simulink model "power_grid"  (R2025a)
settings: Solver=VariableStepAuto  StartTime=0.0  StopTime=10.0  RelTol=1e-3
model workspace (MAT data in the model file):
  HPD_1min = 0
values from neighbouring files (symbols this model uses):
  bus_voltage = 230e3    (= 230000)    [initialise.m]
  wind_farm_power = 150e6    (= 150000000)    [initialise.m]
libraries: spsThreePhasePISectionLineLib x7, spsThreePhaseBreakerLib x7, simulink x6, spsThreePhaseVIMeasurementLib x5, spsLoadFlowBusLib x5, spsThreePhaseSeriesRLCLoadLib x4, spsThreePhaseSourceLib x2, spsWindTurbineInductionGeneratorPhasorTypeLib x1, sps_lib x1
settings Model: Creator=pavan  LastModifiedBy=jamim

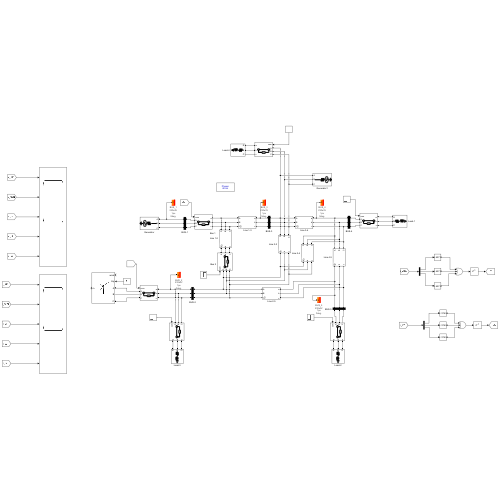
[thumbnail: Simulink's stored preview of the top-level diagram]
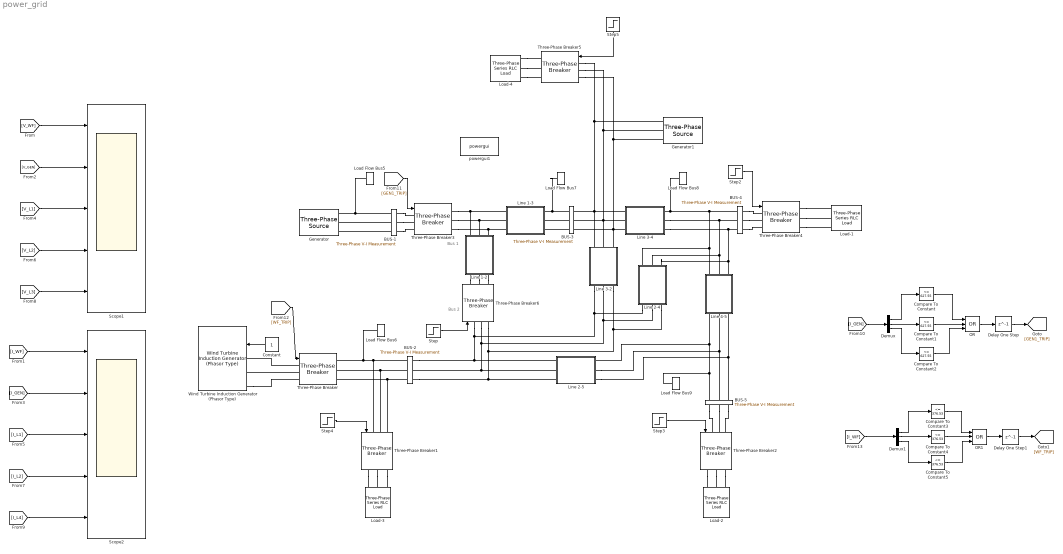
== system power_grid ==
  note: Bus 2
  note: Bus 1
  " Line 1-2" : Subsystem  mask{F=60, SB=100e6, V=230e3, R=0.02, X=0.06, B=0.03}
      mask prompts: F "Frequency"; SB "Base power"; V "Nominal Voltage"; R "Resistance(pu)"; X "Reactance(pu)"; B "Line Charging"
  " Line 1-3" : Subsystem  mask{F=60, SB=100e6, V=230e3, R=0.08, X=0.24, B=0.025}
      mask prompts: F "Frequency"; SB "Base power"; V "Nominal Voltage"; R "Resistance(pu)"; X "Reactance(pu)"; B "Line Charging"
  " Line 2-4" : Subsystem  mask{F=60, SB=100e6, V=230e3, R=0.06, X=0.18, B=0.02}
      mask prompts: F "Frequency"; SB "Base power"; V "Nominal Voltage"; R "Resistance(pu)"; X "Reactance(pu)"; B "Line Charging"
  " Line 2-5" : Subsystem  mask{F=60, SB=100e6, V=230e3, R=0.04, X=0.12, B=0.015}
      mask prompts: F "Frequency"; SB "Base power"; V "Nominal Voltage"; R "Resistance(pu)"; X "Reactance(pu)"; B "Line Charging"
  " Line 3-2" : Subsystem  mask{F=60, SB=100e6, V=230e3, R=0.06, X=0.25, B=0.20}
      mask prompts: F "Frequency"; SB "Base power"; V "Nominal Voltage"; R "Resistance(pu)"; X "Reactance(pu)"; B "Line Charging"
  " Line 3-4" : Subsystem  mask{F=60, SB=100e6, V=230e3, R=0.01, X=0.03, B=0.01}
      mask prompts: F "Frequency"; SB "Base power"; V "Nominal Voltage"; R "Resistance(pu)"; X "Reactance(pu)"; B "Line Charging"
  " Line 4-5" : Subsystem  mask{F=60, SB=100e6, V=230e3, R=0.08, X=0.24, B=0.025}
      mask prompts: F "Frequency"; SB "Base power"; V "Nominal Voltage"; R "Resistance(pu)"; X "Reactance(pu)"; B "Line Charging"
  BUS-1 : spsThreePhaseVIMeasurementLib/Three-Phase V-I Measurement  VoltageMeasurement=phase-to-ground  SetLabelV=on  LabelV=V_GEN  Vpu=off  VpuLL=off  CurrentMeasurement=yes  SetLabelI=on  LabelI=I_GEN  Ipu=off  Pbase=100e6  Vbase=500e3  OutputType=Magnitude  PhasorSimulation=on  PSBequivalent=0
  BUS-2 : spsThreePhaseVIMeasurementLib/Three-Phase V-I Measurement  VoltageMeasurement=phase-to-ground  SetLabelV=on  LabelV=V_WF  Vpu=off  VpuLL=off  CurrentMeasurement=yes  SetLabelI=on  LabelI=I_WF  Ipu=off  Pbase=100e6  Vbase=500e3  OutputType=Magnitude  PhasorSimulation=on  PSBequivalent=0
  BUS-3 : spsThreePhaseVIMeasurementLib/Three-Phase V-I Measurement  VoltageMeasurement=no  SetLabelV=off  LabelV=Vabc  Vpu=off  VpuLL=off  CurrentMeasurement=no  SetLabelI=off  LabelI=Iabc  Ipu=off  Pbase=100e6  Vbase=500e3  OutputType=Complex  PhasorSimulation=on  PSBequivalent=0
  BUS-4 : spsThreePhaseVIMeasurementLib/Three-Phase V-I Measurement  VoltageMeasurement=phase-to-ground  SetLabelV=on  LabelV=V_L1  Vpu=off  VpuLL=off  CurrentMeasurement=yes  SetLabelI=on  LabelI=I_L1  Ipu=off  Pbase=100e6  Vbase=500e3  OutputType=Magnitude  PhasorSimulation=on  PSBequivalent=0
  BUS-5 : spsThreePhaseVIMeasurementLib/Three-Phase V-I Measurement  VoltageMeasurement=phase-to-ground  SetLabelV=on  LabelV=V_L2  Vpu=off  VpuLL=off  CurrentMeasurement=yes  SetLabelI=on  LabelI=I_L2  Ipu=off  Pbase=100e6  Vbase=500e3  OutputType=Magnitude  PhasorSimulation=on  PSBequivalent=0
  Compare To Constant : simulink/Logic and Bit Operations/Compare To Constant  relop=<=  const=627.55  OutDataTypeStr=boolean
  Compare To Constant1 : simulink/Logic and Bit Operations/Compare To Constant  relop=<=  const=627.55  OutDataTypeStr=boolean
  Compare To Constant2 : simulink/Logic and Bit Operations/Compare To Constant  relop=<=  const=627.55  OutDataTypeStr=boolean
  Compare To Constant3 : simulink/Logic and Bit Operations/Compare To Constant  relop=<=  const=376.53  OutDataTypeStr=boolean
  Compare To Constant4 : simulink/Logic and Bit Operations/Compare To Constant  relop=<=  const=376.53  OutDataTypeStr=boolean
  Compare To Constant5 : simulink/Logic and Bit Operations/Compare To Constant  relop=<=  const=376.53  OutDataTypeStr=boolean
  Constant : Constant
  Delay One Step : Delay  DelayLength=1
  Delay One Step1 : Delay  DelayLength=1
  Demux : Demux  Outputs=3
  Demux1 : Demux  Outputs=3
  Generator : spsThreePhaseSourceLib/Three-Phase Source  InternalConnection=Yg  VoltagePhases=off  Voltage=1.06*bus_voltage  PhaseAngle=0  Voltage_phases=[25e3 25e3 25e3]/sqrt(3)  PhaseAngles_phases=[0 -120 +120]  Frequency=60  NonIdealSource=on  SpecifyImpedance=off  Resistance=1e-6  Inductance=0  ShortCircuitLevel=100e6  BaseVoltage=bus_voltage  XRratio=7  BusType=swing  Pref=generator_power  Qref=0  Prefabc=[10e3, 10e3, 10e3]  Qrefabc=[0, 0, 0]  Qmin=-inf  Qmax=inf
  Generator1 : spsThreePhaseSourceLib/Three-Phase Source  InternalConnection=Yg  VoltagePhases=off  Voltage=1.02*bus_voltage  PhaseAngle=0  Voltage_phases=[25e3 25e3 25e3]/sqrt(3)  PhaseAngles_phases=[0 -120 +120]  Frequency=60  NonIdealSource=on  SpecifyImpedance=off  Resistance=1e-6  Inductance=0  ShortCircuitLevel=100e6  BaseVoltage=bus_voltage  XRratio=7  BusType=PV  Pref=generator_power  Qref=0  Prefabc=[10e3, 10e3, 10e3]  Qrefabc=[0, 0, 0]  Qmin=-inf  Qmax=inf
  Load Flow Bus5 : spsLoadFlowBusLib/Load Flow Bus  LConnTagsString=a  Phases=single  Connectors=on one side  ID=BUS_1  Vbase=230e3  Vref=1.06  Vangle=0  VLF=1  VLFb=1  VLFc=1  angleLF=0  angleLFb=0  angleLFc=0
  Load Flow Bus6 : spsLoadFlowBusLib/Load Flow Bus  LConnTagsString=a  Phases=single  Connectors=on one side  ID=BUS_2  Vbase=230e3  Vref=1  Vangle=0  VLF=1  VLFb=1  VLFc=1  angleLF=0  angleLFb=0  angleLFc=0
  Load Flow Bus7 : spsLoadFlowBusLib/Load Flow Bus  LConnTagsString=a  Phases=single  Connectors=on one side  ID=BUS_3  Vbase=230e3  Vref=1  Vangle=0  VLF=1  VLFb=1  VLFc=1  angleLF=0  angleLFb=0  angleLFc=0
  Load Flow Bus8 : spsLoadFlowBusLib/Load Flow Bus  LConnTagsString=a  Phases=single  Connectors=on one side  ID=BUS_4  Vbase=230e3  Vref=1  Vangle=0  VLF=1  VLFb=1  VLFc=1  angleLF=0  angleLFb=0  angleLFc=0
  Load Flow Bus9 : spsLoadFlowBusLib/Load Flow Bus  LConnTagsString=a  Phases=single  Connectors=on one side  ID=BUS_5  Vbase=230e3  Vref=1  Vangle=0  VLF=1  VLFb=1  VLFc=1  angleLF=0  angleLFb=0  angleLFc=0
  Load-1 : spsThreePhaseSeriesRLCLoadLib/Three-Phase Series RLC Load  LConnTagsString=A|B|C  Configuration=Y (grounded)  NominalVoltage=230e3  Vabc=[1e3 1e3 1e3]  Vabcp=[1e3 1e3 1e3]  NominalFrequency=60  UnbalancedPower=off  ActivePower=40e6  InductivePower=20e6  CapacitivePower=0  Pabc=[10e3 9e3 11e3]  QLabc=[100 90 110]  QCabc=[100 90 110]  Pabcp=[10e3 9e3 11e3]  QLabcp=[100 90 110]  QCabcp=[100 90 110]  Measurements=None  LoadType=constant PQ
  Load-2 : spsThreePhaseSeriesRLCLoadLib/Three-Phase Series RLC Load  LConnTagsString=A|B|C  Configuration=Y (grounded)  NominalVoltage=230e3  Vabc=[1e3 1e3 1e3]  Vabcp=[1e3 1e3 1e3]  NominalFrequency=60  UnbalancedPower=off  ActivePower=30e6  InductivePower=15e6  CapacitivePower=0  Pabc=[10e3 9e3 11e3]  QLabc=[100 90 110]  QCabc=[100 90 110]  Pabcp=[10e3 9e3 11e3]  QLabcp=[100 90 110]  QCabcp=[100 90 110]  Measurements=None  LoadType=constant PQ
  Load-3 : spsThreePhaseSeriesRLCLoadLib/Three-Phase Series RLC Load  LConnTagsString=A|B|C  Configuration=Y (grounded)  NominalVoltage=230e3  Vabc=[1e3 1e3 1e3]  Vabcp=[1e3 1e3 1e3]  NominalFrequency=60  UnbalancedPower=off  ActivePower=20e6  InductivePower=10e6  CapacitivePower=0  Pabc=[10e3 9e3 11e3]  QLabc=[100 90 110]  QCabc=[100 90 110]  Pabcp=[10e3 9e3 11e3]  QLabcp=[100 90 110]  QCabcp=[100 90 110]  Measurements=Branch voltages  LoadType=constant PQ
  Load-4 : spsThreePhaseSeriesRLCLoadLib/Three-Phase Series RLC Load  LConnTagsString=A|B|C  Configuration=Y (grounded)  NominalVoltage=230e3  Vabc=[1e3 1e3 1e3]  Vabcp=[1e3 1e3 1e3]  NominalFrequency=60  UnbalancedPower=off  ActivePower=10e6  InductivePower=5e6  CapacitivePower=0  Pabc=[10e3 9e3 11e3]  QLabc=[100 90 110]  QCabc=[100 90 110]  Pabcp=[10e3 9e3 11e3]  QLabcp=[100 90 110]  QCabcp=[100 90 110]  Measurements=None  LoadType=constant PQ
  OR : Logic  Operator=OR  Inputs=3  IconShape=distinctive  AllPortsSameDT=off  OutDataTypeStr=boolean
  OR1 : Logic  Operator=OR  Inputs=3  IconShape=distinctive  AllPortsSameDT=off  OutDataTypeStr=boolean
  Scope1 : Scope  NumInputPorts=5
      settings: ActiveDisplayString=5  Title=Load 3  ActiveDisplayYMinimum=193679.1526589058  ActiveDisplayYMaximum=193679.16399669697
  Scope2 : Scope  NumInputPorts=5
      settings: ActiveDisplayString=5  Title=Load 3  ActiveDisplayYMinimum=171.73759952382511  ActiveDisplayYMaximum=171.84427493175139  DataLoggingVariableName=ScopeData2
  Step{,2..5} (5 alike) : Step  Time=0  SampleTime=0
  Three-Phase Breaker{,1..6} (7 alike) : spsThreePhaseBreakerLib/Three-Phase Breaker  InitialState=closed  SwitchA=on  SwitchB=on  SwitchC=on  SwitchTimes="[1/60  5/60]"  External=on  BreakerResistance=0.01  SnubberResistance=1e6  SnubberCapacitance=inf  Measurements=None
  Wind Turbine Induction Generator (Phasor Type) : spsWindTurbineInductionGeneratorPhasorTypeLib/Wind Turbine Induction Generator (Phasor Type)  ExternalTm=off  nom=[wind_farm_power, 1.04*bus_voltage, 60]  sta=[ 0.004843, 0.1248]  rot=[ 0.004377, 0.1791]  Lm=6.77  mec=[5.04, 0.01, 3]  init="[ -0.01,0,   0,0,0,   0,0,0 ]"  pitch_angle=0  Pmec=1.5e6  wind_base=9  speed_nom=1  P_wind_base=1  K_pitch_gain=[5 25]  pitch_max=45  pitch_rate=2
      settings: LibrarySourceBlock=|
      | sps_lib/Electrical Machines/Wind Turbine
      | Induction Generator
      | (Phasor Type)
  powergui1 : sps_lib/powergui  Priority=1  SimulationMode=Phasor  SampleTime=50e-6  frequency=60  Iterations=50  frequencyindice=60  Pbase=100e6  ErrMax=1e-4  UnitsV=kV  UnitsW=MW  buscounter=0  FunctionMessages=off  echomessages=off  EnableUseOfTLC=off  CurrentSourceSwitches=off  DisableSnubberDevices=off  DisableRonSwitches=off  DisableVfSwitches=off  DisplayEquations=off  AutomaticDiscreteSolvers=off  SolverType=Tustin/Backward Euler (TBE)  Interpol=off  ExternalGateDelay=off  methode=off  Ts=100  x0status=blocks  SPID=on  SwTol=0  HookPort=off  NonlinearTolerance=1e-4  nMaxIteration=100  ContinueOnMaxIteration=off  RestoreLinks=warning  ResistiveCurrentMeasurement=off  Frange=[0:2:500]  Ylog=off  Xlog=on  ShowGrid=off  save=off  variable=ZData  structure=0  ZoomFFT=off  StartTime=0.0  cycles=1  DisplayStyle=1  fundamental=60  FreqAxis=off  MaxFrequency=1000  frequencyindicesteady=1  RmsSteady=1  display=off
  wires:
  Constant/1 -> Wind Turbine Induction Generator (Phasor Type)/2
  [WF_TRIP] -> Three-Phase Breaker/1
  [GEN1_TRIP] -> Three-Phase Breaker3/1
  Step2/1 -> Three-Phase Breaker4/1
  Step3/1 -> Three-Phase Breaker2/1
  Step4/1 -> Three-Phase Breaker1/1
  [V_GEN] -> Scope1/2
  [V_L1] -> Scope1/3
  [V_L2] -> Scope1/4
  [V_L3] -> Scope1/5
  [V_WF] -> Scope1/1
  [I_WF] -> Scope2/1
  [I_GEN] -> Scope2/2
  [I_L1] -> Scope2/3
  [I_L4] -> Scope2/5
  [I_L2] -> Scope2/4
  [I_GEN] -> Demux/1
  Demux/1 -> Compare To Constant/1
  Demux/2 -> Compare To Constant1/1
  Demux/3 -> Compare To Constant2/1
  Compare To Constant/1 -> OR/1
  Compare To Constant1/1 -> OR/2
  Compare To Constant2/1 -> OR/3
  OR/1 -> Delay One Step/1
  Delay One Step/1 -> [GEN1_TRIP]
  Demux1/1 -> Compare To Constant3/1
  OR1/1 -> Delay One Step1/1
  Compare To Constant3/1 -> OR1/1
  Delay One Step1/1 -> [WF_TRIP]
  [I_WF] -> Demux1/1
  Demux1/2 -> Compare To Constant4/1
  Compare To Constant4/1 -> OR1/2
  Demux1/3 -> Compare To Constant5/1
  Compare To Constant5/1 -> OR1/3
  Step/1 -> Three-Phase Breaker6/1
  Step5/1 -> Three-Phase Breaker5/1
  connections:
  Three-Phase Breaker/LConn2 -- Wind Turbine Induction Generator (Phasor Type)/LConn2
  Wind Turbine Induction Generator (Phasor Type)/LConn3 -- Three-Phase Breaker/LConn3
  BUS-3/RConn3 -- Three-Phase Breaker5/LConn3 -- Generator1/RConn3 -- " Line 3-4"/LConn3 -- " Line 3-2"/LConn3
  BUS-3/RConn2 -- Three-Phase Breaker5/LConn2 -- Generator1/RConn2 -- " Line 3-4"/LConn2 -- " Line 3-2"/LConn2
  " Line 1-2"/LConn1 -- Three-Phase Breaker3/RConn1 -- " Line 1-3"/LConn1
  Load Flow Bus5/LConn1 -- BUS-1/LConn1 -- Generator/RConn1
  BUS-3/LConn1 -- Load Flow Bus7/LConn1 -- " Line 1-3"/RConn1
  " Line 1-2"/LConn3 -- Three-Phase Breaker3/RConn3 -- " Line 1-3"/LConn3
  " Line 1-2"/LConn2 -- Three-Phase Breaker3/RConn2 -- " Line 1-3"/LConn2
  BUS-3/RConn1 -- Three-Phase Breaker5/LConn1 -- Generator1/RConn1 -- " Line 3-4"/LConn1 -- " Line 3-2"/LConn1
  BUS-3/LConn2 -- " Line 1-3"/RConn2
  BUS-1/LConn3 -- Generator/RConn3
  BUS-3/LConn3 -- " Line 1-3"/RConn3
  BUS-1/LConn2 -- Generator/RConn2
  Load Flow Bus6/LConn1 -- Three-Phase Breaker1/LConn1 -- BUS-2/LConn1 -- Three-Phase Breaker/RConn1
  BUS-2/LConn2 -- Three-Phase Breaker1/LConn2 -- Three-Phase Breaker/RConn2
  BUS-2/LConn3 -- Three-Phase Breaker1/LConn3 -- Three-Phase Breaker/RConn3
  " Line 3-4"/RConn1 -- Load Flow Bus8/LConn1 -- " Line 2-4"/LConn1 -- " Line 4-5"/LConn1 -- BUS-4/LConn1
  " Line 3-4"/RConn2 -- " Line 2-4"/LConn2 -- " Line 4-5"/LConn2 -- BUS-4/LConn2
  " Line 3-4"/RConn3 -- " Line 2-4"/LConn3 -- " Line 4-5"/LConn3 -- BUS-4/LConn3
  BUS-5/LConn2 -- " Line 2-5"/RConn2 -- " Line 4-5"/RConn2
  BUS-5/LConn3 -- " Line 4-5"/RConn3 -- " Line 2-5"/RConn3
  " Line 2-5"/LConn1 -- BUS-2/RConn1 -- " Line 3-2"/RConn1 -- " Line 2-4"/RConn1 -- Three-Phase Breaker6/LConn1
  " Line 2-4"/RConn3 -- " Line 3-2"/RConn3 -- Three-Phase Breaker6/LConn3 -- " Line 2-5"/LConn3 -- BUS-2/RConn3
  Three-Phase Breaker1/RConn1 -- Load-3/LConn1
  Three-Phase Breaker1/RConn2 -- Load-3/LConn2
  Three-Phase Breaker1/RConn3 -- Load-3/LConn3
  Three-Phase Breaker2/RConn1 -- Load-2/LConn1
  Three-Phase Breaker2/RConn2 -- Load-2/LConn2
  Three-Phase Breaker2/RConn3 -- Load-2/LConn3
  BUS-1/RConn1 -- Three-Phase Breaker3/LConn1
  BUS-1/RConn2 -- Three-Phase Breaker3/LConn2
  BUS-1/RConn3 -- Three-Phase Breaker3/LConn3
  Three-Phase Breaker4/RConn1 -- Load-1/LConn1
  Three-Phase Breaker4/RConn2 -- Load-1/LConn2
  Three-Phase Breaker4/RConn3 -- Load-1/LConn3
  BUS-5/RConn1 -- Three-Phase Breaker2/LConn1
  BUS-5/RConn2 -- Three-Phase Breaker2/LConn2
  BUS-5/RConn3 -- Three-Phase Breaker2/LConn3
  Three-Phase Breaker/LConn1 -- Wind Turbine Induction Generator (Phasor Type)/LConn1
  " Line 1-2"/RConn1 -- Three-Phase Breaker6/RConn1
  " Line 1-2"/RConn2 -- Three-Phase Breaker6/RConn2
  " Line 1-2"/RConn3 -- Three-Phase Breaker6/RConn3
  " Line 3-2"/RConn2 -- Three-Phase Breaker6/LConn2 -- BUS-2/RConn2 -- " Line 2-5"/LConn2 -- " Line 2-4"/RConn2
  BUS-5/LConn1 -- " Line 2-5"/RConn1 -- " Line 4-5"/RConn1 -- Load Flow Bus9/LConn1
  BUS-4/RConn1 -- Three-Phase Breaker4/LConn1
  BUS-4/RConn2 -- Three-Phase Breaker4/LConn2
  BUS-4/RConn3 -- Three-Phase Breaker4/LConn3
  Load-4/LConn1 -- Three-Phase Breaker5/RConn1
  Load-4/LConn3 -- Three-Phase Breaker5/RConn3
  Load-4/LConn2 -- Three-Phase Breaker5/RConn2

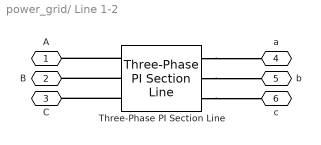
== system power_grid/ Line 1-2 ==
  Three-Phase PI Section Line : spsThreePhasePISectionLineLib/Three-Phase PI Section Line  LConnTagsString=a|b|c  RConnTagsString=A|B|C  Length=floor((3e5)*(sqrt(X*B))/(2*pi*F))  Frequency=F  Resistances=[ (R*(V^2)/SB)/floor((3e5)*(sqrt(X*B))/(2*pi*F)) 3*(R*(V^2)/SB)/floor((3e5)*(sqrt(X*B))/(2*pi*F))]  Inductances=[ (X*(V^2)/SB)/(2*pi*F*floor((3e5)*(sqrt(X*B))/(2*pi*F))) 3*(X*(V^2)/SB)/(2*pi*F*floor((3e5)*(sqrt(X*B))/(2*pi*F)))]  Capacitances=[(B*SB)/((floor((3e5)*(sqrt(X*B))/(2*pi*F)))*2*pi*F*V^2) (3*B*SB)/((floor((3e5)*(sqrt(X*B))/(2*pi*F)))*2*pi*F*V^2)]
  A : PMIOPort  Side=Left
  B : PMIOPort  Port=2  Side=Left
  C : PMIOPort  Port=3  Side=Left
  a : PMIOPort  Port=4  Side=Right
  b : PMIOPort  Port=5  Side=Right
  c : PMIOPort  Port=6  Side=Right
  connections:
  Three-Phase PI Section Line/RConn1 -- a/RConn1
  Three-Phase PI Section Line/LConn3 -- C/RConn1
  Three-Phase PI Section Line/LConn1 -- A/RConn1
  Three-Phase PI Section Line/RConn3 -- c/RConn1
  Three-Phase PI Section Line/RConn2 -- b/RConn1
  Three-Phase PI Section Line/LConn2 -- B/RConn1

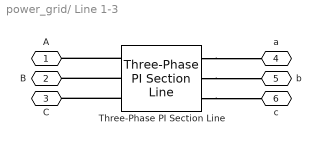
== system power_grid/ Line 1-3 ==
  Three-Phase PI Section Line : spsThreePhasePISectionLineLib/Three-Phase PI Section Line  LConnTagsString=a|b|c  RConnTagsString=A|B|C  Length=floor((3e5)*(sqrt(X*B))/(2*pi*F))  Frequency=F  Resistances=[ (R*(V^2)/SB)/floor((3e5)*(sqrt(X*B))/(2*pi*F)) 3*(R*(V^2)/SB)/floor((3e5)*(sqrt(X*B))/(2*pi*F))]  Inductances=[ (X*(V^2)/SB)/(2*pi*F*floor((3e5)*(sqrt(X*B))/(2*pi*F))) 3*(X*(V^2)/SB)/(2*pi*F*floor((3e5)*(sqrt(X*B))/(2*pi*F)))]  Capacitances=[(B*SB)/((floor((3e5)*(sqrt(X*B))/(2*pi*F)))*2*pi*F*V^2) (3*B*SB)/((floor((3e5)*(sqrt(X*B))/(2*pi*F)))*2*pi*F*V^2)]
  A : PMIOPort  Side=Left
  B : PMIOPort  Port=2  Side=Left
  C : PMIOPort  Port=3  Side=Left
  a : PMIOPort  Port=4  Side=Right
  b : PMIOPort  Port=5  Side=Right
  c : PMIOPort  Port=6  Side=Right
  connections:
  Three-Phase PI Section Line/LConn2 -- B/RConn1
  Three-Phase PI Section Line/RConn2 -- b/RConn1
  Three-Phase PI Section Line/RConn3 -- c/RConn1
  Three-Phase PI Section Line/LConn1 -- A/RConn1
  Three-Phase PI Section Line/LConn3 -- C/RConn1
  Three-Phase PI Section Line/RConn1 -- a/RConn1

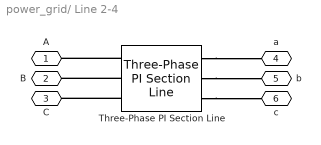
== system power_grid/ Line 2-4 ==
  Three-Phase PI Section Line : spsThreePhasePISectionLineLib/Three-Phase PI Section Line  LConnTagsString=a|b|c  RConnTagsString=A|B|C  Length=floor((3e5)*(sqrt(X*B))/(2*pi*F))  Frequency=F  Resistances=[ (R*(V^2)/SB)/floor((3e5)*(sqrt(X*B))/(2*pi*F)) 3*(R*(V^2)/SB)/floor((3e5)*(sqrt(X*B))/(2*pi*F))]  Inductances=[ (X*(V^2)/SB)/(2*pi*F*floor((3e5)*(sqrt(X*B))/(2*pi*F))) 3*(X*(V^2)/SB)/(2*pi*F*floor((3e5)*(sqrt(X*B))/(2*pi*F)))]  Capacitances=[(B*SB)/((floor((3e5)*(sqrt(X*B))/(2*pi*F)))*2*pi*F*V^2) (3*B*SB)/((floor((3e5)*(sqrt(X*B))/(2*pi*F)))*2*pi*F*V^2)]
  A : PMIOPort  Side=Left
  B : PMIOPort  Port=2  Side=Left
  C : PMIOPort  Port=3  Side=Left
  a : PMIOPort  Port=4  Side=Right
  b : PMIOPort  Port=5  Side=Right
  c : PMIOPort  Port=6  Side=Right
  connections:
  Three-Phase PI Section Line/RConn1 -- a/RConn1
  Three-Phase PI Section Line/LConn3 -- C/RConn1
  Three-Phase PI Section Line/LConn1 -- A/RConn1
  Three-Phase PI Section Line/RConn3 -- c/RConn1
  Three-Phase PI Section Line/RConn2 -- b/RConn1
  Three-Phase PI Section Line/LConn2 -- B/RConn1

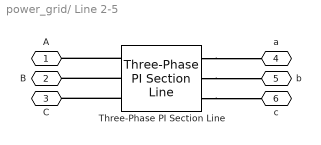
== system power_grid/ Line 2-5 ==
  Three-Phase PI Section Line : spsThreePhasePISectionLineLib/Three-Phase PI Section Line  LConnTagsString=a|b|c  RConnTagsString=A|B|C  Length=floor((3e5)*(sqrt(X*B))/(2*pi*F))  Frequency=F  Resistances=[ (R*(V^2)/SB)/floor((3e5)*(sqrt(X*B))/(2*pi*F)) 3*(R*(V^2)/SB)/floor((3e5)*(sqrt(X*B))/(2*pi*F))]  Inductances=[ (X*(V^2)/SB)/(2*pi*F*floor((3e5)*(sqrt(X*B))/(2*pi*F))) 3*(X*(V^2)/SB)/(2*pi*F*floor((3e5)*(sqrt(X*B))/(2*pi*F)))]  Capacitances=[(B*SB)/((floor((3e5)*(sqrt(X*B))/(2*pi*F)))*2*pi*F*V^2) (3*B*SB)/((floor((3e5)*(sqrt(X*B))/(2*pi*F)))*2*pi*F*V^2)]
  A : PMIOPort  Side=Left
  B : PMIOPort  Port=2  Side=Left
  C : PMIOPort  Port=3  Side=Left
  a : PMIOPort  Port=4  Side=Right
  b : PMIOPort  Port=5  Side=Right
  c : PMIOPort  Port=6  Side=Right
  connections:
  Three-Phase PI Section Line/LConn2 -- B/RConn1
  Three-Phase PI Section Line/RConn2 -- b/RConn1
  Three-Phase PI Section Line/RConn3 -- c/RConn1
  Three-Phase PI Section Line/LConn1 -- A/RConn1
  Three-Phase PI Section Line/LConn3 -- C/RConn1
  Three-Phase PI Section Line/RConn1 -- a/RConn1

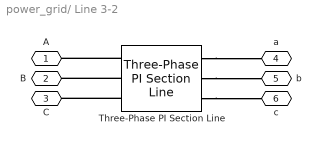
== system power_grid/ Line 3-2 ==
  Three-Phase PI Section Line : spsThreePhasePISectionLineLib/Three-Phase PI Section Line  LConnTagsString=a|b|c  RConnTagsString=A|B|C  Length=floor((3e5)*(sqrt(X*B))/(2*pi*F))  Frequency=F  Resistances=[ (R*(V^2)/SB)/floor((3e5)*(sqrt(X*B))/(2*pi*F)) 3*(R*(V^2)/SB)/floor((3e5)*(sqrt(X*B))/(2*pi*F))]  Inductances=[ (X*(V^2)/SB)/(2*pi*F*floor((3e5)*(sqrt(X*B))/(2*pi*F))) 3*(X*(V^2)/SB)/(2*pi*F*floor((3e5)*(sqrt(X*B))/(2*pi*F)))]  Capacitances=[(B*SB)/((floor((3e5)*(sqrt(X*B))/(2*pi*F)))*2*pi*F*V^2) (3*B*SB)/((floor((3e5)*(sqrt(X*B))/(2*pi*F)))*2*pi*F*V^2)]
  A : PMIOPort  Side=Left
  B : PMIOPort  Port=2  Side=Left
  C : PMIOPort  Port=3  Side=Left
  a : PMIOPort  Port=4  Side=Right
  b : PMIOPort  Port=5  Side=Right
  c : PMIOPort  Port=6  Side=Right
  connections:
  Three-Phase PI Section Line/LConn2 -- B/RConn1
  Three-Phase PI Section Line/RConn2 -- b/RConn1
  Three-Phase PI Section Line/RConn3 -- c/RConn1
  Three-Phase PI Section Line/LConn1 -- A/RConn1
  Three-Phase PI Section Line/LConn3 -- C/RConn1
  Three-Phase PI Section Line/RConn1 -- a/RConn1

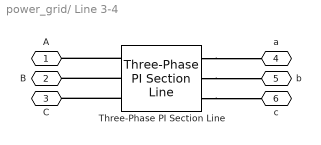
== system power_grid/ Line 3-4 ==
  Three-Phase PI Section Line : spsThreePhasePISectionLineLib/Three-Phase PI Section Line  LConnTagsString=a|b|c  RConnTagsString=A|B|C  Length=floor((3e5)*(sqrt(X*B))/(2*pi*F))  Frequency=F  Resistances=[ (R*(V^2)/SB)/floor((3e5)*(sqrt(X*B))/(2*pi*F)) 3*(R*(V^2)/SB)/floor((3e5)*(sqrt(X*B))/(2*pi*F))]  Inductances=[ (X*(V^2)/SB)/(2*pi*F*floor((3e5)*(sqrt(X*B))/(2*pi*F))) 3*(X*(V^2)/SB)/(2*pi*F*floor((3e5)*(sqrt(X*B))/(2*pi*F)))]  Capacitances=[(B*SB)/((floor((3e5)*(sqrt(X*B))/(2*pi*F)))*2*pi*F*V^2) (3*B*SB)/((floor((3e5)*(sqrt(X*B))/(2*pi*F)))*2*pi*F*V^2)]
  A : PMIOPort  Side=Left
  B : PMIOPort  Port=2  Side=Left
  C : PMIOPort  Port=3  Side=Left
  a : PMIOPort  Port=4  Side=Right
  b : PMIOPort  Port=5  Side=Right
  c : PMIOPort  Port=6  Side=Right
  connections:
  Three-Phase PI Section Line/RConn1 -- a/RConn1
  Three-Phase PI Section Line/LConn3 -- C/RConn1
  Three-Phase PI Section Line/LConn1 -- A/RConn1
  Three-Phase PI Section Line/RConn3 -- c/RConn1
  Three-Phase PI Section Line/RConn2 -- b/RConn1
  Three-Phase PI Section Line/LConn2 -- B/RConn1

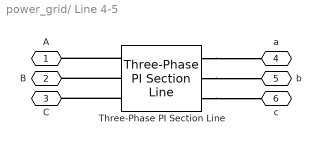
== system power_grid/ Line 4-5 ==
  Three-Phase PI Section Line : spsThreePhasePISectionLineLib/Three-Phase PI Section Line  LConnTagsString=a|b|c  RConnTagsString=A|B|C  Length=floor((3e5)*(sqrt(X*B))/(2*pi*F))  Frequency=F  Resistances=[ (R*(V^2)/SB)/floor((3e5)*(sqrt(X*B))/(2*pi*F)) 3*(R*(V^2)/SB)/floor((3e5)*(sqrt(X*B))/(2*pi*F))]  Inductances=[ (X*(V^2)/SB)/(2*pi*F*floor((3e5)*(sqrt(X*B))/(2*pi*F))) 3*(X*(V^2)/SB)/(2*pi*F*floor((3e5)*(sqrt(X*B))/(2*pi*F)))]  Capacitances=[(B*SB)/((floor((3e5)*(sqrt(X*B))/(2*pi*F)))*2*pi*F*V^2) (3*B*SB)/((floor((3e5)*(sqrt(X*B))/(2*pi*F)))*2*pi*F*V^2)]
  A : PMIOPort  Side=Left
  B : PMIOPort  Port=2  Side=Left
  C : PMIOPort  Port=3  Side=Left
  a : PMIOPort  Port=4  Side=Right
  b : PMIOPort  Port=5  Side=Right
  c : PMIOPort  Port=6  Side=Right
  connections:
  Three-Phase PI Section Line/LConn2 -- B/RConn1
  Three-Phase PI Section Line/RConn2 -- b/RConn1
  Three-Phase PI Section Line/RConn3 -- c/RConn1
  Three-Phase PI Section Line/LConn1 -- A/RConn1
  Three-Phase PI Section Line/LConn3 -- C/RConn1
  Three-Phase PI Section Line/RConn1 -- a/RConn1
